simulink model "PulsePairProc_x4"  (Simulink 6.4)
settings: Solver=ode45  StartTime=0.0  StopTime=40000/12e6  RelTol=1e-3
libraries: xbsIndex_r4 x1049, simulink x4, dspsrcs4 x1
(part 3 of 8)

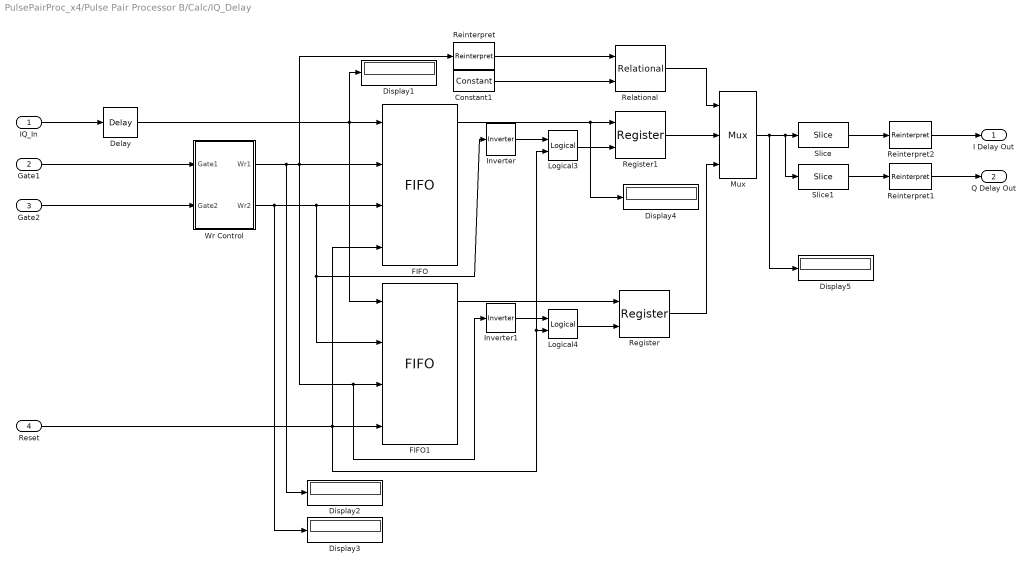
== system PulsePairProc_x4/Pulse Pair Processor B/Calc/IQ_Delay ==
  IQ_In : Inport
  Gate1 : Inport  Port=2
  Gate2 : Inport  Port=3
  Reset : Inport  Port=4
  Constant1 : xbsIndex_r4/Constant  arith_type=Unsigned  const=1  n_bits=1  bin_pt=0  explicit_period=off  period=1  equ=P=C  opselect=C  inp2=PCIN>>17  opr=+  inp1=P  carry=CIN  dbl_ovrd=off  block_type=constant
      settings: block_version=8.2
  Delay : xbsIndex_r4/Delay  en=off  latency=2  dbl_ovrd=off  reg_retiming=off  block_type=delay
      settings: infoedit=Hardware notes: A delay line is a chain, each link of which is an SRL16 followed by a flip-flop. If register retiming is enabled, the delay line is a chain of flip-flops.  block_version=8.2
  Display{1..5} (5 alike) : Display
  FIFO : xbsIndex_r4/FIFO  depth=1K  percent_nbits=1  rst=on  en=off  dbl_ovrd=off  mem_type=Block RAM  block_type=fifo
      settings: block_version=8.2
  FIFO1 : xbsIndex_r4/FIFO  depth=1K  percent_nbits=1  rst=on  en=off  dbl_ovrd=off  mem_type=Block RAM  block_type=fifo
      settings: block_version=8.2
  Inverter : xbsIndex_r4/Inverter  en=off  latency=1  dbl_ovrd=off  block_type=inv
      settings: block_version=8.2
  Inverter1 : xbsIndex_r4/Inverter  en=off  latency=1  dbl_ovrd=off  block_type=inv
      settings: block_version=8.2
  Logical3 : xbsIndex_r4/Logical  logical_function=OR  inputs=2  en=off  latency=0  precision=Full  arith_type=Unsigned  n_bits=16  bin_pt=0  align_bp=on  dbl_ovrd=off  block_type=logical
      settings: block_version=8.2
  Logical4 : xbsIndex_r4/Logical  logical_function=OR  inputs=2  en=off  latency=0  precision=Full  arith_type=Unsigned  n_bits=16  bin_pt=0  align_bp=on  dbl_ovrd=off  block_type=logical
      settings: block_version=8.2
  Mux : xbsIndex_r4/Mux  inputs=2  en=off  latency=0  precision=Full  arith_type=Unsigned  n_bits=16  bin_pt=14  quantization=Truncate  overflow=Wrap  dbl_ovrd=off  block_type=mux
      settings: block_version=8.2
  Register : xbsIndex_r4/Register  init=0  rst=on  en=off  dbl_ovrd=off  block_type=register
      settings: block_version=8.2
  Register1 : xbsIndex_r4/Register  init=0  rst=on  en=off  dbl_ovrd=off  block_type=register
      settings: block_version=8.2
  Reinterpret : xbsIndex_r4/Reinterpret  force_arith_type=on  arith_type=Unsigned  force_bin_pt=off  bin_pt=0  block_type=reinterpret
      settings: infoedit="Changes signal type without altering the binary representation.   You can changed the signal between signed and unsigned, and relocate the binary point.<P><P>Hardware notes: In hardware this block costs nothing.<P><P>Example:  Suppose the input is 6 bits wide, signed, with 2 fractional bits, and the output is forced to unsigned with 0 fractional bits.  Then an input of -2.0 (1110.00 in binary 2's complement) becomes an output of 56 (111000 in binary)."  block_version=8.2
  Reinterpret1 : xbsIndex_r4/Reinterpret  force_arith_type=on  arith_type="Signed  (2's comp)"  force_bin_pt=on  bin_pt=15  block_type=reinterpret
      settings: infoedit="Changes signal type without altering the binary representation.   You can changed the signal between signed and unsigned, and relocate the binary point.<P><P>Hardware notes: In hardware this block costs nothing.<P><P>Example:  Suppose the input is 6 bits wide, signed, with 2 fractional bits, and the output is forced to unsigned with 0 fractional bits.  Then an input of -2.0 (1110.00 in binary 2's complement) becomes an output of 56 (111000 in binary)."  block_version=8.2
  Reinterpret2 : xbsIndex_r4/Reinterpret  force_arith_type=on  arith_type="Signed  (2's comp)"  force_bin_pt=on  bin_pt=15  block_type=reinterpret
      settings: infoedit="Changes signal type without altering the binary representation.   You can changed the signal between signed and unsigned, and relocate the binary point.<P><P>Hardware notes: In hardware this block costs nothing.<P><P>Example:  Suppose the input is 6 bits wide, signed, with 2 fractional bits, and the output is forced to unsigned with 0 fractional bits.  Then an input of -2.0 (1110.00 in binary 2's complement) becomes an output of 56 (111000 in binary)."  block_version=8.2
  Relational : xbsIndex_r4/Relational  mode=a=b  en=off  latency=2  dbl_ovrd=off  block_type=relational
      settings: block_version=8.2
  Slice : xbsIndex_r4/Slice  nbits=16  boolean_output=off  mode=Upper Bit Location + Width  bit1=0  base1=MSB of Input  bit0=0  base0=LSB of Input  dbl_ovrd=off  block_type=slice
      settings: infoedit="Extracts a given range of bits from each input sample and presents it at the output.  The output type is ordinarily unsigned with binary point at zero, but can be Boolean when the slice is one bit wide.<P><P>Hardware notes: In hardware this block costs nothing."  block_version=8.2
  Slice1 : xbsIndex_r4/Slice  nbits=16  boolean_output=off  mode=Lower Bit Location + Width  bit1=0  base1=MSB of Input  bit0=0  base0=LSB of Input  dbl_ovrd=off  block_type=slice
      settings: infoedit="Extracts a given range of bits from each input sample and presents it at the output.  The output type is ordinarily unsigned with binary point at zero, but can be Boolean when the slice is one bit wide.<P><P>Hardware notes: In hardware this block costs nothing."  block_version=8.2
  Wr Control : Subsystem
  I Delay Out : Outport
  Q Delay Out : Outport  Port=2
  wires:
  IQ_In/1 -> Delay/1
  Reset/1 -> FIFO/4, FIFO1/4, Logical4/2, Logical3/2
  FIFO1/1 -> Register/1
  FIFO/1 -> Register1/1, Display4/1
  Register1/1 -> Mux/2
  Register/1 -> Mux/3
  Relational/1 -> Mux/1
  Constant1/1 -> Relational/2
  Reinterpret/1 -> Relational/1
  Delay/1 -> FIFO1/1, FIFO/1, Display1/1
  Logical3/1 -> Register1/2
  Logical4/1 -> Register/2
  Inverter1/1 -> Logical4/1
  Inverter/1 -> Logical3/1
  Mux/1 -> Slice/1, Slice1/1, Display5/1
  Slice/1 -> Reinterpret2/1
  Slice1/1 -> Reinterpret1/1
  Reinterpret1/1 -> Q Delay Out/1
  Reinterpret2/1 -> I Delay Out/1
  Wr Control/1(Wr1) -> FIFO/2, Reinterpret/1, FIFO1/3, Inverter1/1, Display2/1
  Wr Control/2(Wr2) -> FIFO/3, FIFO1/2, Inverter/1, Display3/1
  Gate1/1 -> Wr Control/1(Gate1)
  Gate2/1 -> Wr Control/2(Gate2)

== system PulsePairProc_x4/Pulse Pair Processor B/Calc/I^2+Q^2 ==
  I : Inport
  Q : Inport  Port=2
  AddSub : xbsIndex_r4/AddSub  mode=Addition  use_carryin=off  use_carryout=off  en=off  latency=1  precision=User Defined  arith_type=Unsigned  n_bits=32  bin_pt=32  quantization="Round  (unbiased: +/- Inf)"  overflow=Flag as error  dbl_ovrd=off  use_behavioral_HDL=off  pipelined=on  use_rpm=on  block_type=addsub
      settings: block_version=8.2
  Mult : xbsIndex_r4/Mult  precision=User Defined  arith_type=Unsigned  n_bits=32  bin_pt=32  quantization="Round  (unbiased: +/- Inf)"  overflow=Flag as error  en=off  latency=1  dbl_ovrd=off  use_behavioral_HDL=off  use_embedded=on  optimum_pipeline=off  use_rpm=on  placement_style=Rectangular shape  pipeline=on  block_type=mult
      settings: infoedit=Hardware notes: To use the internal pipeline stage of the dedicated multiplier you must select 'Pipeline for maximum performance'.  block_version=8.2
  Mult1 : xbsIndex_r4/Mult  precision=User Defined  arith_type=Unsigned  n_bits=32  bin_pt=32  quantization="Round  (unbiased: +/- Inf)"  overflow=Flag as error  en=off  latency=1  dbl_ovrd=off  use_behavioral_HDL=off  use_embedded=on  optimum_pipeline=off  use_rpm=on  placement_style=Rectangular shape  pipeline=on  block_type=mult
      settings: infoedit=Hardware notes: To use the internal pipeline stage of the dedicated multiplier you must select 'Pipeline for maximum performance'.  block_version=8.2
  P : Outport
  wires:
  Mult/1 -> AddSub/1
  Mult1/1 -> AddSub/2
  I/1 -> Mult/1, Mult/2
  Q/1 -> Mult1/1, Mult1/2
  AddSub/1 -> P/1

== system PulsePairProc_x4/Pulse Pair Processor B/Calc/Q*Id1-I*Qd1 ==
  Q : Inport
  I Delay 1 : Inport  Port=2
  I : Inport  Port=3
  Q Delay 1 : Inport  Port=4
  AddSub2 : xbsIndex_r4/AddSub  mode=Subtraction  use_carryin=off  use_carryout=off  en=off  latency=1  precision=User Defined  arith_type="Signed  (2's comp)"  n_bits=32  bin_pt=31  quantization="Round  (unbiased: +/- Inf)"  overflow=Flag as error  dbl_ovrd=off  use_behavioral_HDL=off  pipelined=on  use_rpm=on  block_type=addsub
      settings: block_version=8.2
  Mult4 : xbsIndex_r4/Mult  precision=User Defined  arith_type="Signed  (2's comp)"  n_bits=32  bin_pt=31  quantization="Round  (unbiased: +/- Inf)"  overflow=Saturate  en=off  latency=1  dbl_ovrd=off  use_behavioral_HDL=off  use_embedded=on  optimum_pipeline=off  use_rpm=on  placement_style=Rectangular shape  pipeline=on  block_type=mult
      settings: infoedit=Hardware notes: To use the internal pipeline stage of the dedicated multiplier you must select 'Pipeline for maximum performance'.  block_version=8.2
  Mult5 : xbsIndex_r4/Mult  precision=User Defined  arith_type="Signed  (2's comp)"  n_bits=32  bin_pt=31  quantization="Round  (unbiased: +/- Inf)"  overflow=Saturate  en=off  latency=1  dbl_ovrd=off  use_behavioral_HDL=off  use_embedded=on  optimum_pipeline=off  use_rpm=on  placement_style=Rectangular shape  pipeline=on  block_type=mult
      settings: infoedit=Hardware notes: To use the internal pipeline stage of the dedicated multiplier you must select 'Pipeline for maximum performance'.  block_version=8.2
  B : Outport
  wires:
  Mult4/1 -> AddSub2/1
  Mult5/1 -> AddSub2/2
  Q/1 -> Mult4/1
  I Delay 1/1 -> Mult4/2
  AddSub2/1 -> B/1
  I/1 -> Mult5/1
  Q Delay 1/1 -> Mult5/2

== system PulsePairProc_x4/Pulse Pair Processor B/Sum/A Avg ==
  A_Data_In : Inport
  M : Inport  Port=2
  N : Inport  Port=3
  Gate 1 : Inport  Port=4
  Gate 2 : Inport  Port=5
  Reset : Inport  Port=6
  Avg. A 1 : Subsystem
  Avg. A 2 : Subsystem
  A1 : Outport
  A2 : Outport  Port=2
  ABP G1 : Outport  Port=3
  ABP G2 : Outport  Port=4
  wires:
  A_Data_In/1 -> Avg. A 1/1(In), Avg. A 2/1(In)
  M/1 -> Avg. A 1/2(M), Avg. A 2/2(M)
  N/1 -> Avg. A 1/3(N), Avg. A 2/3(N)
  Avg. A 1/1(Out) -> A1/1
  Gate 1/1 -> Avg. A 1/4(Gate)
  Avg. A 2/1(Out) -> A2/1
  Gate 2/1 -> Avg. A 2/4(Gate)
  Avg. A 1/2(A,B,P Gate 1) -> ABP G1/1
  Avg. A 2/2(A,B,P Gate 1) -> ABP G2/1
  Reset/1 -> Avg. A 1/5(Reset), Avg. A 2/5(Reset)

== system PulsePairProc_x4/Pulse Pair Processor B/Sum/B Avg ==
  B_Data_In : Inport
  M : Inport  Port=2
  N : Inport  Port=3
  Gate 1 : Inport  Port=4
  Gate 2 : Inport  Port=5
  Reset : Inport  Port=6
  Avg. B 1 : Subsystem
  Avg. B 2 : Subsystem
  B1 : Outport
  B2 : Outport  Port=2
  wires:
  B_Data_In/1 -> Avg. B 1/1(In), Avg. B 2/1(In)
  M/1 -> Avg. B 1/2(M), Avg. B 2/2(M)
  N/1 -> Avg. B 1/3(N), Avg. B 2/3(N)
  Avg. B 1/1(Out) -> B1/1
  Gate 1/1 -> Avg. B 1/4(Gate)
  Avg. B 2/1(Out) -> B2/1
  Gate 2/1 -> Avg. B 2/4(Gate)
  Reset/1 -> Avg. B 1/5(Reset), Avg. B 2/5(Reset)

== system PulsePairProc_x4/Pulse Pair Processor B/Sum/Error Check ==
  Gate_1_In : Inport
  Gate_2_In : Inport  Port=2
  M_Reg : Inport  Port=3
  Counter : xbsIndex_r4/Counter  cnt_type=Free Running  cnt_to=Inf  operation=Up  start_count=0  cnt_by_val=1  arith_type=Unsigned  n_bits=10  bin_pt=0  load_pin=off  rst=on  en=on  explicit_period=on  period=1/12e6  dbl_ovrd=off  use_behavioral_HDL=off  use_rpm=off  block_type=counter
      settings: block_version=8.2
  Counter1 : xbsIndex_r4/Counter  cnt_type=Free Running  cnt_to=Inf  operation=Up  start_count=0  cnt_by_val=1  arith_type=Unsigned  n_bits=10  bin_pt=0  load_pin=off  rst=on  en=on  explicit_period=on  period=1/12e6  dbl_ovrd=off  use_behavioral_HDL=off  use_rpm=off  block_type=counter
      settings: block_version=8.2
  Delay{,1..3} (4 alike) : xbsIndex_r4/Delay  en=off  latency=1  dbl_ovrd=off  reg_retiming=off  block_type=delay
      settings: infoedit=Hardware notes: A delay line is a chain, each link of which is an SRL16 followed by a flip-flop. If register retiming is enabled, the delay line is a chain of flip-flops.  block_version=8.2
  Inverter : xbsIndex_r4/Inverter  en=off  latency=0  dbl_ovrd=off  block_type=inv
      settings: block_version=8.2
  Inverter1 : xbsIndex_r4/Inverter  en=off  latency=0  dbl_ovrd=off  block_type=inv
      settings: block_version=8.2
  Logical : xbsIndex_r4/Logical  logical_function=OR  inputs=2  en=off  latency=0  precision=Full  arith_type=Unsigned  n_bits=16  bin_pt=0  align_bp=on  dbl_ovrd=off  block_type=logical
      settings: block_version=8.2
  Register : xbsIndex_r4/Register  init=0  rst=off  en=on  dbl_ovrd=off  block_type=register
      settings: block_version=8.2
  Register1 : xbsIndex_r4/Register  init=0  rst=on  en=on  dbl_ovrd=off  block_type=register
      settings: block_version=8.2
  Register2 : xbsIndex_r4/Register  init=0  rst=off  en=on  dbl_ovrd=off  block_type=register
      settings: block_version=8.2
  Register3 : xbsIndex_r4/Register  init=0  rst=on  en=on  dbl_ovrd=off  block_type=register
      settings: block_version=8.2
  Relational : xbsIndex_r4/Relational  mode=a!=b  en=on  latency=1  dbl_ovrd=off  block_type=relational
      settings: block_version=8.2
  Relational1 : xbsIndex_r4/Relational  mode=a!=b  en=on  latency=1  dbl_ovrd=off  block_type=relational
      settings: block_version=8.2
  Sync Error : Outport
  wires:
  Inverter/1 -> Counter/1, Register/2, Delay/1, Register1/1
  Counter/1 -> Register/1
  Register/1 -> Relational/1
  Gate_1_In/1 -> Inverter/1, Counter/2, Delay1/1
  Delay/1 -> Register1/2
  Register1/1 -> Relational/3
  Delay1/1 -> Register1/3
  Inverter1/1 -> Counter1/1, Register2/2, Delay2/1, Register3/1
  Counter1/1 -> Register2/1
  Register2/1 -> Relational1/1
  Gate_2_In/1 -> Inverter1/1, Counter1/2, Delay3/1
  M_Reg/1 -> Relational1/2, Relational/2
  Delay2/1 -> Register3/2
  Register3/1 -> Relational1/3
  Delay3/1 -> Register3/3
  Relational/1 -> Logical/1
  Relational1/1 -> Logical/2
  Logical/1 -> Sync Error/1

== system PulsePairProc_x4/Pulse Pair Processor B/Sum/IQ Selector ==
  IQ Data : Inport
  IQ Gate 1 : Inport  Port=2
  IQ Gate 2 : Inport  Port=3
  IQ Index : Inport  Port=4
  IQ Length : Inport  Port=5
  Counter : xbsIndex_r4/Counter  cnt_type=Count Limited  cnt_to=1023  operation=Up  start_count=0  cnt_by_val=1  arith_type=Unsigned  n_bits=10  bin_pt=0  load_pin=off  rst=on  en=on  explicit_period=on  period=1/12e6  dbl_ovrd=off  use_behavioral_HDL=off  use_rpm=off  block_type=counter
      settings: block_version=8.2
  Counter1 : xbsIndex_r4/Counter  cnt_type=Count Limited  cnt_to=1023  operation=Up  start_count=0  cnt_by_val=1  arith_type=Unsigned  n_bits=10  bin_pt=0  load_pin=off  rst=on  en=on  explicit_period=on  period=1/12e6  dbl_ovrd=off  use_behavioral_HDL=off  use_rpm=off  block_type=counter
      settings: block_version=8.2
  Delay{,1..3} (4 alike) : xbsIndex_r4/Delay  en=off  latency=3  dbl_ovrd=off  reg_retiming=off  block_type=delay
      settings: infoedit=Hardware notes: A delay line is a chain, each link of which is an SRL16 followed by a flip-flop. If register retiming is enabled, the delay line is a chain of flip-flops.  block_version=8.2
  Inverter : xbsIndex_r4/Inverter  en=off  latency=0  dbl_ovrd=off  block_type=inv
      settings: block_version=8.2
  Inverter1 : xbsIndex_r4/Inverter  en=off  latency=0  dbl_ovrd=off  block_type=inv
      settings: block_version=8.2
  Inverter2 : xbsIndex_r4/Inverter  en=off  latency=0  dbl_ovrd=off  block_type=inv
      settings: block_version=8.2
  Inverter4 : xbsIndex_r4/Inverter  en=off  latency=1  dbl_ovrd=off  block_type=inv
      settings: block_version=8.2
  Logical{,1..3} (4 alike) : xbsIndex_r4/Logical  logical_function=OR  inputs=2  en=off  latency=0  precision=Full  arith_type=Unsigned  n_bits=16  bin_pt=0  align_bp=on  dbl_ovrd=off  block_type=logical
      settings: block_version=8.2
  Logical4 : xbsIndex_r4/Logical  logical_function=AND  inputs=2  en=off  latency=0  precision=Full  arith_type=Unsigned  n_bits=16  bin_pt=0  align_bp=on  dbl_ovrd=off  block_type=logical
      settings: block_version=8.2
  Logical5 : xbsIndex_r4/Logical  logical_function=AND  inputs=2  en=off  latency=0  precision=Full  arith_type=Unsigned  n_bits=16  bin_pt=0  align_bp=on  dbl_ovrd=off  block_type=logical
      settings: block_version=8.2
  Register1 : xbsIndex_r4/Register  init=0  rst=on  en=off  dbl_ovrd=off  block_type=register
      settings: block_version=8.2
  Relational : xbsIndex_r4/Relational  mode=a>b  en=on  latency=1  dbl_ovrd=off  block_type=relational
      settings: block_version=8.2
  Relational1 : xbsIndex_r4/Relational  mode=a<b  en=on  latency=1  dbl_ovrd=off  block_type=relational
      settings: block_version=8.2
  IQ Out : Outport
  IQ Gate 1 Out : Outport  Port=2
  IQ Gate 2 Out : Outport  Port=3
  wires:
  Counter/1 -> Relational/1
  IQ Index/1 -> Relational/2
  Inverter/1 -> Counter/1, Delay/1
  Inverter1/1 -> Counter1/1
  Relational/1 -> Inverter1/1, Counter1/2, Relational1/3
  Counter1/1 -> Relational1/1
  Relational1/1 -> Inverter2/1
  IQ Data/1 -> Register1/1
  Register1/1 -> Delay2/1
  Logical/1 -> Inverter/1, Counter/2, Relational/3
  IQ Gate 2/1 -> Logical/2, Logical5/2
  IQ Gate 1/1 -> Logical/1, Logical4/2
  Logical1/1 -> Register1/2, Inverter4/1
  Inverter2/1 -> Logical1/2
  Delay/1 -> Logical1/1
  IQ Length/1 -> Relational1/2
  Logical2/1 -> IQ Gate 1 Out/1
  Delay1/1 -> Logical2/1
  Delay2/1 -> IQ Out/1
  Inverter4/1 -> Logical4/1, Logical5/1
  Logical4/1 -> Delay1/1, Logical2/2
  Logical3/1 -> IQ Gate 2 Out/1
  Delay3/1 -> Logical3/1
  Logical5/1 -> Delay3/1, Logical3/2

== system PulsePairProc_x4/Pulse Pair Processor B/Sum/P Avg ==
  P_Data_In : Inport
  M : Inport  Port=2
  N : Inport  Port=3
  Gate 1 : Inport  Port=4
  Gate 2 : Inport  Port=5
  Reset : Inport  Port=6
  Avg. P 1 : Subsystem
  Avg. P 2 : Subsystem
  P1 : Outport
  P2 : Outport  Port=2
  wires:
  P_Data_In/1 -> Avg. P 1/1(In), Avg. P 2/1(In)
  M/1 -> Avg. P 1/2(M), Avg. P 2/2(M)
  N/1 -> Avg. P 1/3(N), Avg. P 2/3(N)
  Avg. P 1/1(Out) -> P1/1
  Gate 1/1 -> Avg. P 1/4(Gate)
  Avg. P 2/1(Out) -> P2/1
  Gate 2/1 -> Avg. P 2/4(Gate)
  Reset/1 -> Avg. P 1/5(Reset), Avg. P 2/5(Reset)

== system PulsePairProc_x4/Pulse Pair Processor C/Calc/I*Id1+Q*Qd1 ==
  I : Inport
  I Delay 1 : Inport  Port=2
  Q : Inport  Port=3
  Q Delay 1 : Inport  Port=4
  AddSub1 : xbsIndex_r4/AddSub  mode=Addition  use_carryin=off  use_carryout=off  en=off  latency=1  precision=User Defined  arith_type="Signed  (2's comp)"  n_bits=32  bin_pt=31  quantization="Round  (unbiased: +/- Inf)"  overflow=Flag as error  dbl_ovrd=off  use_behavioral_HDL=off  pipelined=on  use_rpm=on  block_type=addsub
      settings: block_version=8.2
  Mult2 : xbsIndex_r4/Mult  precision=User Defined  arith_type="Signed  (2's comp)"  n_bits=32  bin_pt=31  quantization="Round  (unbiased: +/- Inf)"  overflow=Saturate  en=off  latency=1  dbl_ovrd=off  use_behavioral_HDL=off  use_embedded=on  optimum_pipeline=off  use_rpm=on  placement_style=Rectangular shape  pipeline=on  block_type=mult
      settings: infoedit=Hardware notes: To use the internal pipeline stage of the dedicated multiplier you must select 'Pipeline for maximum performance'.  block_version=8.2
  Mult3 : xbsIndex_r4/Mult  precision=User Defined  arith_type="Signed  (2's comp)"  n_bits=32  bin_pt=31  quantization="Round  (unbiased: +/- Inf)"  overflow=Saturate  en=off  latency=1  dbl_ovrd=off  use_behavioral_HDL=off  use_embedded=on  optimum_pipeline=off  use_rpm=on  placement_style=Rectangular shape  pipeline=on  block_type=mult
      settings: infoedit=Hardware notes: To use the internal pipeline stage of the dedicated multiplier you must select 'Pipeline for maximum performance'.  block_version=8.2
  A : Outport
  wires:
  Mult2/1 -> AddSub1/1
  Mult3/1 -> AddSub1/2
  I/1 -> Mult2/1
  I Delay 1/1 -> Mult2/2
  AddSub1/1 -> A/1
  Q/1 -> Mult3/1
  Q Delay 1/1 -> Mult3/2

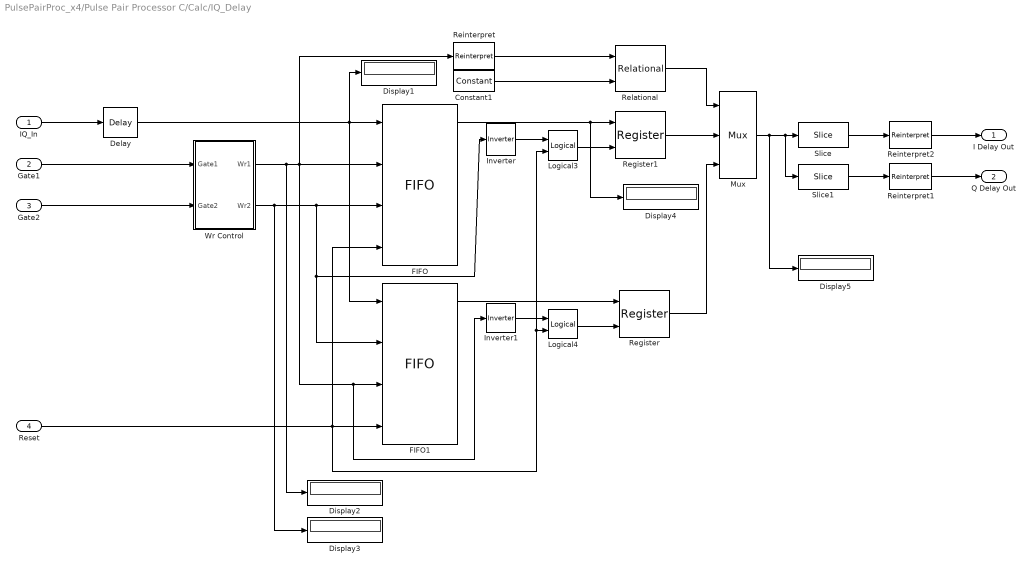
== system PulsePairProc_x4/Pulse Pair Processor C/Calc/IQ_Delay ==
  IQ_In : Inport
  Gate1 : Inport  Port=2
  Gate2 : Inport  Port=3
  Reset : Inport  Port=4
  Constant1 : xbsIndex_r4/Constant  arith_type=Unsigned  const=1  n_bits=1  bin_pt=0  explicit_period=off  period=1  equ=P=C  opselect=C  inp2=PCIN>>17  opr=+  inp1=P  carry=CIN  dbl_ovrd=off  block_type=constant
      settings: block_version=8.2
  Delay : xbsIndex_r4/Delay  en=off  latency=2  dbl_ovrd=off  reg_retiming=off  block_type=delay
      settings: infoedit=Hardware notes: A delay line is a chain, each link of which is an SRL16 followed by a flip-flop. If register retiming is enabled, the delay line is a chain of flip-flops.  block_version=8.2
  Display{1..5} (5 alike) : Display
  FIFO : xbsIndex_r4/FIFO  depth=1K  percent_nbits=1  rst=on  en=off  dbl_ovrd=off  mem_type=Block RAM  block_type=fifo
      settings: block_version=8.2
  FIFO1 : xbsIndex_r4/FIFO  depth=1K  percent_nbits=1  rst=on  en=off  dbl_ovrd=off  mem_type=Block RAM  block_type=fifo
      settings: block_version=8.2
  Inverter : xbsIndex_r4/Inverter  en=off  latency=1  dbl_ovrd=off  block_type=inv
      settings: block_version=8.2
  Inverter1 : xbsIndex_r4/Inverter  en=off  latency=1  dbl_ovrd=off  block_type=inv
      settings: block_version=8.2
  Logical3 : xbsIndex_r4/Logical  logical_function=OR  inputs=2  en=off  latency=0  precision=Full  arith_type=Unsigned  n_bits=16  bin_pt=0  align_bp=on  dbl_ovrd=off  block_type=logical
      settings: block_version=8.2
  Logical4 : xbsIndex_r4/Logical  logical_function=OR  inputs=2  en=off  latency=0  precision=Full  arith_type=Unsigned  n_bits=16  bin_pt=0  align_bp=on  dbl_ovrd=off  block_type=logical
      settings: block_version=8.2
  Mux : xbsIndex_r4/Mux  inputs=2  en=off  latency=0  precision=Full  arith_type=Unsigned  n_bits=16  bin_pt=14  quantization=Truncate  overflow=Wrap  dbl_ovrd=off  block_type=mux
      settings: block_version=8.2
  Register : xbsIndex_r4/Register  init=0  rst=on  en=off  dbl_ovrd=off  block_type=register
      settings: block_version=8.2
  Register1 : xbsIndex_r4/Register  init=0  rst=on  en=off  dbl_ovrd=off  block_type=register
      settings: block_version=8.2
  Reinterpret : xbsIndex_r4/Reinterpret  force_arith_type=on  arith_type=Unsigned  force_bin_pt=off  bin_pt=0  block_type=reinterpret
      settings: infoedit="Changes signal type without altering the binary representation.   You can changed the signal between signed and unsigned, and relocate the binary point.<P><P>Hardware notes: In hardware this block costs nothing.<P><P>Example:  Suppose the input is 6 bits wide, signed, with 2 fractional bits, and the output is forced to unsigned with 0 fractional bits.  Then an input of -2.0 (1110.00 in binary 2's complement) becomes an output of 56 (111000 in binary)."  block_version=8.2
  Reinterpret1 : xbsIndex_r4/Reinterpret  force_arith_type=on  arith_type="Signed  (2's comp)"  force_bin_pt=on  bin_pt=15  block_type=reinterpret
      settings: infoedit="Changes signal type without altering the binary representation.   You can changed the signal between signed and unsigned, and relocate the binary point.<P><P>Hardware notes: In hardware this block costs nothing.<P><P>Example:  Suppose the input is 6 bits wide, signed, with 2 fractional bits, and the output is forced to unsigned with 0 fractional bits.  Then an input of -2.0 (1110.00 in binary 2's complement) becomes an output of 56 (111000 in binary)."  block_version=8.2
  Reinterpret2 : xbsIndex_r4/Reinterpret  force_arith_type=on  arith_type="Signed  (2's comp)"  force_bin_pt=on  bin_pt=15  block_type=reinterpret
      settings: infoedit="Changes signal type without altering the binary representation.   You can changed the signal between signed and unsigned, and relocate the binary point.<P><P>Hardware notes: In hardware this block costs nothing.<P><P>Example:  Suppose the input is 6 bits wide, signed, with 2 fractional bits, and the output is forced to unsigned with 0 fractional bits.  Then an input of -2.0 (1110.00 in binary 2's complement) becomes an output of 56 (111000 in binary)."  block_version=8.2
  Relational : xbsIndex_r4/Relational  mode=a=b  en=off  latency=2  dbl_ovrd=off  block_type=relational
      settings: block_version=8.2
  Slice : xbsIndex_r4/Slice  nbits=16  boolean_output=off  mode=Upper Bit Location + Width  bit1=0  base1=MSB of Input  bit0=0  base0=LSB of Input  dbl_ovrd=off  block_type=slice
      settings: infoedit="Extracts a given range of bits from each input sample and presents it at the output.  The output type is ordinarily unsigned with binary point at zero, but can be Boolean when the slice is one bit wide.<P><P>Hardware notes: In hardware this block costs nothing."  block_version=8.2
  Slice1 : xbsIndex_r4/Slice  nbits=16  boolean_output=off  mode=Lower Bit Location + Width  bit1=0  base1=MSB of Input  bit0=0  base0=LSB of Input  dbl_ovrd=off  block_type=slice
      settings: infoedit="Extracts a given range of bits from each input sample and presents it at the output.  The output type is ordinarily unsigned with binary point at zero, but can be Boolean when the slice is one bit wide.<P><P>Hardware notes: In hardware this block costs nothing."  block_version=8.2
  Wr Control : Subsystem
  I Delay Out : Outport
  Q Delay Out : Outport  Port=2
  wires:
  IQ_In/1 -> Delay/1
  Reset/1 -> FIFO/4, FIFO1/4, Logical4/2, Logical3/2
  FIFO1/1 -> Register/1
  FIFO/1 -> Register1/1, Display4/1
  Register1/1 -> Mux/2
  Register/1 -> Mux/3
  Relational/1 -> Mux/1
  Constant1/1 -> Relational/2
  Reinterpret/1 -> Relational/1
  Delay/1 -> FIFO1/1, FIFO/1, Display1/1
  Logical3/1 -> Register1/2
  Logical4/1 -> Register/2
  Inverter1/1 -> Logical4/1
  Inverter/1 -> Logical3/1
  Mux/1 -> Slice/1, Slice1/1, Display5/1
  Slice/1 -> Reinterpret2/1
  Slice1/1 -> Reinterpret1/1
  Reinterpret1/1 -> Q Delay Out/1
  Reinterpret2/1 -> I Delay Out/1
  Wr Control/1(Wr1) -> FIFO/2, Reinterpret/1, FIFO1/3, Inverter1/1, Display2/1
  Wr Control/2(Wr2) -> FIFO/3, FIFO1/2, Inverter/1, Display3/1
  Gate1/1 -> Wr Control/1(Gate1)
  Gate2/1 -> Wr Control/2(Gate2)

== system PulsePairProc_x4/Pulse Pair Processor C/Calc/I^2+Q^2 ==
  I : Inport
  Q : Inport  Port=2
  AddSub : xbsIndex_r4/AddSub  mode=Addition  use_carryin=off  use_carryout=off  en=off  latency=1  precision=User Defined  arith_type=Unsigned  n_bits=32  bin_pt=32  quantization="Round  (unbiased: +/- Inf)"  overflow=Flag as error  dbl_ovrd=off  use_behavioral_HDL=off  pipelined=on  use_rpm=on  block_type=addsub
      settings: block_version=8.2
  Mult : xbsIndex_r4/Mult  precision=User Defined  arith_type=Unsigned  n_bits=32  bin_pt=32  quantization="Round  (unbiased: +/- Inf)"  overflow=Flag as error  en=off  latency=1  dbl_ovrd=off  use_behavioral_HDL=off  use_embedded=on  optimum_pipeline=off  use_rpm=on  placement_style=Rectangular shape  pipeline=on  block_type=mult
      settings: infoedit=Hardware notes: To use the internal pipeline stage of the dedicated multiplier you must select 'Pipeline for maximum performance'.  block_version=8.2
  Mult1 : xbsIndex_r4/Mult  precision=User Defined  arith_type=Unsigned  n_bits=32  bin_pt=32  quantization="Round  (unbiased: +/- Inf)"  overflow=Flag as error  en=off  latency=1  dbl_ovrd=off  use_behavioral_HDL=off  use_embedded=on  optimum_pipeline=off  use_rpm=on  placement_style=Rectangular shape  pipeline=on  block_type=mult
      settings: infoedit=Hardware notes: To use the internal pipeline stage of the dedicated multiplier you must select 'Pipeline for maximum performance'.  block_version=8.2
  P : Outport
  wires:
  Mult/1 -> AddSub/1
  Mult1/1 -> AddSub/2
  I/1 -> Mult/1, Mult/2
  Q/1 -> Mult1/1, Mult1/2
  AddSub/1 -> P/1

== system PulsePairProc_x4/Pulse Pair Processor C/Calc/Q*Id1-I*Qd1 ==
  Q : Inport
  I Delay 1 : Inport  Port=2
  I : Inport  Port=3
  Q Delay 1 : Inport  Port=4
  AddSub2 : xbsIndex_r4/AddSub  mode=Subtraction  use_carryin=off  use_carryout=off  en=off  latency=1  precision=User Defined  arith_type="Signed  (2's comp)"  n_bits=32  bin_pt=31  quantization="Round  (unbiased: +/- Inf)"  overflow=Flag as error  dbl_ovrd=off  use_behavioral_HDL=off  pipelined=on  use_rpm=on  block_type=addsub
      settings: block_version=8.2
  Mult4 : xbsIndex_r4/Mult  precision=User Defined  arith_type="Signed  (2's comp)"  n_bits=32  bin_pt=31  quantization="Round  (unbiased: +/- Inf)"  overflow=Saturate  en=off  latency=1  dbl_ovrd=off  use_behavioral_HDL=off  use_embedded=on  optimum_pipeline=off  use_rpm=on  placement_style=Rectangular shape  pipeline=on  block_type=mult
      settings: infoedit=Hardware notes: To use the internal pipeline stage of the dedicated multiplier you must select 'Pipeline for maximum performance'.  block_version=8.2
  Mult5 : xbsIndex_r4/Mult  precision=User Defined  arith_type="Signed  (2's comp)"  n_bits=32  bin_pt=31  quantization="Round  (unbiased: +/- Inf)"  overflow=Saturate  en=off  latency=1  dbl_ovrd=off  use_behavioral_HDL=off  use_embedded=on  optimum_pipeline=off  use_rpm=on  placement_style=Rectangular shape  pipeline=on  block_type=mult
      settings: infoedit=Hardware notes: To use the internal pipeline stage of the dedicated multiplier you must select 'Pipeline for maximum performance'.  block_version=8.2
  B : Outport
  wires:
  Mult4/1 -> AddSub2/1
  Mult5/1 -> AddSub2/2
  Q/1 -> Mult4/1
  I Delay 1/1 -> Mult4/2
  AddSub2/1 -> B/1
  I/1 -> Mult5/1
  Q Delay 1/1 -> Mult5/2

== system PulsePairProc_x4/Pulse Pair Processor C/Sum/A Avg ==
  A_Data_In : Inport
  M : Inport  Port=2
  N : Inport  Port=3
  Gate 1 : Inport  Port=4
  Gate 2 : Inport  Port=5
  Reset : Inport  Port=6
  Avg. A 1 : Subsystem
  Avg. A 2 : Subsystem
  A1 : Outport
  A2 : Outport  Port=2
  ABP G1 : Outport  Port=3
  ABP G2 : Outport  Port=4
  wires:
  A_Data_In/1 -> Avg. A 1/1(In), Avg. A 2/1(In)
  M/1 -> Avg. A 1/2(M), Avg. A 2/2(M)
  N/1 -> Avg. A 1/3(N), Avg. A 2/3(N)
  Avg. A 1/1(Out) -> A1/1
  Gate 1/1 -> Avg. A 1/4(Gate)
  Avg. A 2/1(Out) -> A2/1
  Gate 2/1 -> Avg. A 2/4(Gate)
  Avg. A 1/2(A,B,P Gate 1) -> ABP G1/1
  Avg. A 2/2(A,B,P Gate 1) -> ABP G2/1
  Reset/1 -> Avg. A 1/5(Reset), Avg. A 2/5(Reset)

== system PulsePairProc_x4/Pulse Pair Processor C/Sum/B Avg ==
  B_Data_In : Inport
  M : Inport  Port=2
  N : Inport  Port=3
  Gate 1 : Inport  Port=4
  Gate 2 : Inport  Port=5
  Reset : Inport  Port=6
  Avg. B 1 : Subsystem
  Avg. B 2 : Subsystem
  B1 : Outport
  B2 : Outport  Port=2
  wires:
  B_Data_In/1 -> Avg. B 1/1(In), Avg. B 2/1(In)
  M/1 -> Avg. B 1/2(M), Avg. B 2/2(M)
  N/1 -> Avg. B 1/3(N), Avg. B 2/3(N)
  Avg. B 1/1(Out) -> B1/1
  Gate 1/1 -> Avg. B 1/4(Gate)
  Avg. B 2/1(Out) -> B2/1
  Gate 2/1 -> Avg. B 2/4(Gate)
  Reset/1 -> Avg. B 1/5(Reset), Avg. B 2/5(Reset)

== system PulsePairProc_x4/Pulse Pair Processor C/Sum/Error Check ==
  Gate_1_In : Inport
  Gate_2_In : Inport  Port=2
  M_Reg : Inport  Port=3
  Counter : xbsIndex_r4/Counter  cnt_type=Free Running  cnt_to=Inf  operation=Up  start_count=0  cnt_by_val=1  arith_type=Unsigned  n_bits=10  bin_pt=0  load_pin=off  rst=on  en=on  explicit_period=on  period=1/12e6  dbl_ovrd=off  use_behavioral_HDL=off  use_rpm=off  block_type=counter
      settings: block_version=8.2
  Counter1 : xbsIndex_r4/Counter  cnt_type=Free Running  cnt_to=Inf  operation=Up  start_count=0  cnt_by_val=1  arith_type=Unsigned  n_bits=10  bin_pt=0  load_pin=off  rst=on  en=on  explicit_period=on  period=1/12e6  dbl_ovrd=off  use_behavioral_HDL=off  use_rpm=off  block_type=counter
      settings: block_version=8.2
  Delay{,1..3} (4 alike) : xbsIndex_r4/Delay  en=off  latency=1  dbl_ovrd=off  reg_retiming=off  block_type=delay
      settings: infoedit=Hardware notes: A delay line is a chain, each link of which is an SRL16 followed by a flip-flop. If register retiming is enabled, the delay line is a chain of flip-flops.  block_version=8.2
  Inverter : xbsIndex_r4/Inverter  en=off  latency=0  dbl_ovrd=off  block_type=inv
      settings: block_version=8.2
  Inverter1 : xbsIndex_r4/Inverter  en=off  latency=0  dbl_ovrd=off  block_type=inv
      settings: block_version=8.2
  Logical : xbsIndex_r4/Logical  logical_function=OR  inputs=2  en=off  latency=0  precision=Full  arith_type=Unsigned  n_bits=16  bin_pt=0  align_bp=on  dbl_ovrd=off  block_type=logical
      settings: block_version=8.2
  Register : xbsIndex_r4/Register  init=0  rst=off  en=on  dbl_ovrd=off  block_type=register
      settings: block_version=8.2
  Register1 : xbsIndex_r4/Register  init=0  rst=on  en=on  dbl_ovrd=off  block_type=register
      settings: block_version=8.2
  Register2 : xbsIndex_r4/Register  init=0  rst=off  en=on  dbl_ovrd=off  block_type=register
      settings: block_version=8.2
  Register3 : xbsIndex_r4/Register  init=0  rst=on  en=on  dbl_ovrd=off  block_type=register
      settings: block_version=8.2
  Relational : xbsIndex_r4/Relational  mode=a!=b  en=on  latency=1  dbl_ovrd=off  block_type=relational
      settings: block_version=8.2
  Relational1 : xbsIndex_r4/Relational  mode=a!=b  en=on  latency=1  dbl_ovrd=off  block_type=relational
      settings: block_version=8.2
  Sync Error : Outport
  wires:
  Inverter/1 -> Counter/1, Register/2, Delay/1, Register1/1
  Counter/1 -> Register/1
  Register/1 -> Relational/1
  Gate_1_In/1 -> Inverter/1, Counter/2, Delay1/1
  Delay/1 -> Register1/2
  Register1/1 -> Relational/3
  Delay1/1 -> Register1/3
  Inverter1/1 -> Counter1/1, Register2/2, Delay2/1, Register3/1
  Counter1/1 -> Register2/1
  Register2/1 -> Relational1/1
  Gate_2_In/1 -> Inverter1/1, Counter1/2, Delay3/1
  M_Reg/1 -> Relational1/2, Relational/2
  Delay2/1 -> Register3/2
  Register3/1 -> Relational1/3
  Delay3/1 -> Register3/3
  Relational/1 -> Logical/1
  Relational1/1 -> Logical/2
  Logical/1 -> Sync Error/1

== system PulsePairProc_x4/Pulse Pair Processor C/Sum/IQ Selector ==
  IQ Data : Inport
  IQ Gate 1 : Inport  Port=2
  IQ Gate 2 : Inport  Port=3
  IQ Index : Inport  Port=4
  IQ Length : Inport  Port=5
  Counter : xbsIndex_r4/Counter  cnt_type=Count Limited  cnt_to=1023  operation=Up  start_count=0  cnt_by_val=1  arith_type=Unsigned  n_bits=10  bin_pt=0  load_pin=off  rst=on  en=on  explicit_period=on  period=1/12e6  dbl_ovrd=off  use_behavioral_HDL=off  use_rpm=off  block_type=counter
      settings: block_version=8.2
  Counter1 : xbsIndex_r4/Counter  cnt_type=Count Limited  cnt_to=1023  operation=Up  start_count=0  cnt_by_val=1  arith_type=Unsigned  n_bits=10  bin_pt=0  load_pin=off  rst=on  en=on  explicit_period=on  period=1/12e6  dbl_ovrd=off  use_behavioral_HDL=off  use_rpm=off  block_type=counter
      settings: block_version=8.2
  Delay{,1..3} (4 alike) : xbsIndex_r4/Delay  en=off  latency=3  dbl_ovrd=off  reg_retiming=off  block_type=delay
      settings: infoedit=Hardware notes: A delay line is a chain, each link of which is an SRL16 followed by a flip-flop. If register retiming is enabled, the delay line is a chain of flip-flops.  block_version=8.2
  Inverter : xbsIndex_r4/Inverter  en=off  latency=0  dbl_ovrd=off  block_type=inv
      settings: block_version=8.2
  Inverter1 : xbsIndex_r4/Inverter  en=off  latency=0  dbl_ovrd=off  block_type=inv
      settings: block_version=8.2
  Inverter2 : xbsIndex_r4/Inverter  en=off  latency=0  dbl_ovrd=off  block_type=inv
      settings: block_version=8.2
  Inverter4 : xbsIndex_r4/Inverter  en=off  latency=1  dbl_ovrd=off  block_type=inv
      settings: block_version=8.2
  Logical{,1..3} (4 alike) : xbsIndex_r4/Logical  logical_function=OR  inputs=2  en=off  latency=0  precision=Full  arith_type=Unsigned  n_bits=16  bin_pt=0  align_bp=on  dbl_ovrd=off  block_type=logical
      settings: block_version=8.2
  Logical4 : xbsIndex_r4/Logical  logical_function=AND  inputs=2  en=off  latency=0  precision=Full  arith_type=Unsigned  n_bits=16  bin_pt=0  align_bp=on  dbl_ovrd=off  block_type=logical
      settings: block_version=8.2
  Logical5 : xbsIndex_r4/Logical  logical_function=AND  inputs=2  en=off  latency=0  precision=Full  arith_type=Unsigned  n_bits=16  bin_pt=0  align_bp=on  dbl_ovrd=off  block_type=logical
      settings: block_version=8.2
  Register1 : xbsIndex_r4/Register  init=0  rst=on  en=off  dbl_ovrd=off  block_type=register
      settings: block_version=8.2
  Relational : xbsIndex_r4/Relational  mode=a>b  en=on  latency=1  dbl_ovrd=off  block_type=relational
      settings: block_version=8.2
  Relational1 : xbsIndex_r4/Relational  mode=a<b  en=on  latency=1  dbl_ovrd=off  block_type=relational
      settings: block_version=8.2
  IQ Out : Outport
  IQ Gate 1 Out : Outport  Port=2
  IQ Gate 2 Out : Outport  Port=3
  wires:
  Counter/1 -> Relational/1
  IQ Index/1 -> Relational/2
  Inverter/1 -> Counter/1, Delay/1
  Inverter1/1 -> Counter1/1
  Relational/1 -> Inverter1/1, Counter1/2, Relational1/3
  Counter1/1 -> Relational1/1
  Relational1/1 -> Inverter2/1
  IQ Data/1 -> Register1/1
  Register1/1 -> Delay2/1
  Logical/1 -> Inverter/1, Counter/2, Relational/3
  IQ Gate 2/1 -> Logical/2, Logical5/2
  IQ Gate 1/1 -> Logical/1, Logical4/2
  Logical1/1 -> Register1/2, Inverter4/1
  Inverter2/1 -> Logical1/2
  Delay/1 -> Logical1/1
  IQ Length/1 -> Relational1/2
  Logical2/1 -> IQ Gate 1 Out/1
  Delay1/1 -> Logical2/1
  Delay2/1 -> IQ Out/1
  Inverter4/1 -> Logical4/1, Logical5/1
  Logical4/1 -> Delay1/1, Logical2/2
  Logical3/1 -> IQ Gate 2 Out/1
  Delay3/1 -> Logical3/1
  Logical5/1 -> Delay3/1, Logical3/2

== system PulsePairProc_x4/Pulse Pair Processor C/Sum/P Avg ==
  P_Data_In : Inport
  M : Inport  Port=2
  N : Inport  Port=3
  Gate 1 : Inport  Port=4
  Gate 2 : Inport  Port=5
  Reset : Inport  Port=6
  Avg. P 1 : Subsystem
  Avg. P 2 : Subsystem
  P1 : Outport
  P2 : Outport  Port=2
  wires:
  P_Data_In/1 -> Avg. P 1/1(In), Avg. P 2/1(In)
  M/1 -> Avg. P 1/2(M), Avg. P 2/2(M)
  N/1 -> Avg. P 1/3(N), Avg. P 2/3(N)
  Avg. P 1/1(Out) -> P1/1
  Gate 1/1 -> Avg. P 1/4(Gate)
  Avg. P 2/1(Out) -> P2/1
  Gate 2/1 -> Avg. P 2/4(Gate)
  Reset/1 -> Avg. P 1/5(Reset), Avg. P 2/5(Reset)

== system PulsePairProc_x4/Pulse Pair Processor D/Calc/I*Id1+Q*Qd1 ==
  I : Inport
  I Delay 1 : Inport  Port=2
  Q : Inport  Port=3
  Q Delay 1 : Inport  Port=4
  AddSub1 : xbsIndex_r4/AddSub  mode=Addition  use_carryin=off  use_carryout=off  en=off  latency=1  precision=User Defined  arith_type="Signed  (2's comp)"  n_bits=32  bin_pt=31  quantization="Round  (unbiased: +/- Inf)"  overflow=Flag as error  dbl_ovrd=off  use_behavioral_HDL=off  pipelined=on  use_rpm=on  block_type=addsub
      settings: block_version=8.2
  Mult2 : xbsIndex_r4/Mult  precision=User Defined  arith_type="Signed  (2's comp)"  n_bits=32  bin_pt=31  quantization="Round  (unbiased: +/- Inf)"  overflow=Saturate  en=off  latency=1  dbl_ovrd=off  use_behavioral_HDL=off  use_embedded=on  optimum_pipeline=off  use_rpm=on  placement_style=Rectangular shape  pipeline=on  block_type=mult
      settings: infoedit=Hardware notes: To use the internal pipeline stage of the dedicated multiplier you must select 'Pipeline for maximum performance'.  block_version=8.2
  Mult3 : xbsIndex_r4/Mult  precision=User Defined  arith_type="Signed  (2's comp)"  n_bits=32  bin_pt=31  quantization="Round  (unbiased: +/- Inf)"  overflow=Saturate  en=off  latency=1  dbl_ovrd=off  use_behavioral_HDL=off  use_embedded=on  optimum_pipeline=off  use_rpm=on  placement_style=Rectangular shape  pipeline=on  block_type=mult
      settings: infoedit=Hardware notes: To use the internal pipeline stage of the dedicated multiplier you must select 'Pipeline for maximum performance'.  block_version=8.2
  A : Outport
  wires:
  Mult2/1 -> AddSub1/1
  Mult3/1 -> AddSub1/2
  I/1 -> Mult2/1
  I Delay 1/1 -> Mult2/2
  AddSub1/1 -> A/1
  Q/1 -> Mult3/1
  Q Delay 1/1 -> Mult3/2

== system PulsePairProc_x4/Pulse Pair Processor D/Calc/IQ_Delay ==
  IQ_In : Inport
  Gate1 : Inport  Port=2
  Gate2 : Inport  Port=3
  Reset : Inport  Port=4
  Constant1 : xbsIndex_r4/Constant  arith_type=Unsigned  const=1  n_bits=1  bin_pt=0  explicit_period=off  period=1  equ=P=C  opselect=C  inp2=PCIN>>17  opr=+  inp1=P  carry=CIN  dbl_ovrd=off  block_type=constant
      settings: block_version=8.2
  Delay : xbsIndex_r4/Delay  en=off  latency=2  dbl_ovrd=off  reg_retiming=off  block_type=delay
      settings: infoedit=Hardware notes: A delay line is a chain, each link of which is an SRL16 followed by a flip-flop. If register retiming is enabled, the delay line is a chain of flip-flops.  block_version=8.2
  Display{1..5} (5 alike) : Display
  FIFO : xbsIndex_r4/FIFO  depth=1K  percent_nbits=1  rst=on  en=off  dbl_ovrd=off  mem_type=Block RAM  block_type=fifo
      settings: block_version=8.2
  FIFO1 : xbsIndex_r4/FIFO  depth=1K  percent_nbits=1  rst=on  en=off  dbl_ovrd=off  mem_type=Block RAM  block_type=fifo
      settings: block_version=8.2
  Inverter : xbsIndex_r4/Inverter  en=off  latency=1  dbl_ovrd=off  block_type=inv
      settings: block_version=8.2
  Inverter1 : xbsIndex_r4/Inverter  en=off  latency=1  dbl_ovrd=off  block_type=inv
      settings: block_version=8.2
  Logical3 : xbsIndex_r4/Logical  logical_function=OR  inputs=2  en=off  latency=0  precision=Full  arith_type=Unsigned  n_bits=16  bin_pt=0  align_bp=on  dbl_ovrd=off  block_type=logical
      settings: block_version=8.2
  Logical4 : xbsIndex_r4/Logical  logical_function=OR  inputs=2  en=off  latency=0  precision=Full  arith_type=Unsigned  n_bits=16  bin_pt=0  align_bp=on  dbl_ovrd=off  block_type=logical
      settings: block_version=8.2
  Mux : xbsIndex_r4/Mux  inputs=2  en=off  latency=0  precision=Full  arith_type=Unsigned  n_bits=16  bin_pt=14  quantization=Truncate  overflow=Wrap  dbl_ovrd=off  block_type=mux
      settings: block_version=8.2
  Register : xbsIndex_r4/Register  init=0  rst=on  en=off  dbl_ovrd=off  block_type=register
      settings: block_version=8.2
  Register1 : xbsIndex_r4/Register  init=0  rst=on  en=off  dbl_ovrd=off  block_type=register
      settings: block_version=8.2
  Reinterpret : xbsIndex_r4/Reinterpret  force_arith_type=on  arith_type=Unsigned  force_bin_pt=off  bin_pt=0  block_type=reinterpret
      settings: infoedit="Changes signal type without altering the binary representation.   You can changed the signal between signed and unsigned, and relocate the binary point.<P><P>Hardware notes: In hardware this block costs nothing.<P><P>Example:  Suppose the input is 6 bits wide, signed, with 2 fractional bits, and the output is forced to unsigned with 0 fractional bits.  Then an input of -2.0 (1110.00 in binary 2's complement) becomes an output of 56 (111000 in binary)."  block_version=8.2
  Reinterpret1 : xbsIndex_r4/Reinterpret  force_arith_type=on  arith_type="Signed  (2's comp)"  force_bin_pt=on  bin_pt=15  block_type=reinterpret
      settings: infoedit="Changes signal type without altering the binary representation.   You can changed the signal between signed and unsigned, and relocate the binary point.<P><P>Hardware notes: In hardware this block costs nothing.<P><P>Example:  Suppose the input is 6 bits wide, signed, with 2 fractional bits, and the output is forced to unsigned with 0 fractional bits.  Then an input of -2.0 (1110.00 in binary 2's complement) becomes an output of 56 (111000 in binary)."  block_version=8.2
  Reinterpret2 : xbsIndex_r4/Reinterpret  force_arith_type=on  arith_type="Signed  (2's comp)"  force_bin_pt=on  bin_pt=15  block_type=reinterpret
      settings: infoedit="Changes signal type without altering the binary representation.   You can changed the signal between signed and unsigned, and relocate the binary point.<P><P>Hardware notes: In hardware this block costs nothing.<P><P>Example:  Suppose the input is 6 bits wide, signed, with 2 fractional bits, and the output is forced to unsigned with 0 fractional bits.  Then an input of -2.0 (1110.00 in binary 2's complement) becomes an output of 56 (111000 in binary)."  block_version=8.2
  Relational : xbsIndex_r4/Relational  mode=a=b  en=off  latency=2  dbl_ovrd=off  block_type=relational
      settings: block_version=8.2
  Slice : xbsIndex_r4/Slice  nbits=16  boolean_output=off  mode=Upper Bit Location + Width  bit1=0  base1=MSB of Input  bit0=0  base0=LSB of Input  dbl_ovrd=off  block_type=slice
      settings: infoedit="Extracts a given range of bits from each input sample and presents it at the output.  The output type is ordinarily unsigned with binary point at zero, but can be Boolean when the slice is one bit wide.<P><P>Hardware notes: In hardware this block costs nothing."  block_version=8.2
  Slice1 : xbsIndex_r4/Slice  nbits=16  boolean_output=off  mode=Lower Bit Location + Width  bit1=0  base1=MSB of Input  bit0=0  base0=LSB of Input  dbl_ovrd=off  block_type=slice
      settings: infoedit="Extracts a given range of bits from each input sample and presents it at the output.  The output type is ordinarily unsigned with binary point at zero, but can be Boolean when the slice is one bit wide.<P><P>Hardware notes: In hardware this block costs nothing."  block_version=8.2
  Wr Control : Subsystem
  I Delay Out : Outport
  Q Delay Out : Outport  Port=2
  wires:
  IQ_In/1 -> Delay/1
  Reset/1 -> FIFO/4, FIFO1/4, Logical4/2, Logical3/2
  FIFO1/1 -> Register/1
  FIFO/1 -> Register1/1, Display4/1
  Register1/1 -> Mux/2
  Register/1 -> Mux/3
  Relational/1 -> Mux/1
  Constant1/1 -> Relational/2
  Reinterpret/1 -> Relational/1
  Delay/1 -> FIFO1/1, FIFO/1, Display1/1
  Logical3/1 -> Register1/2
  Logical4/1 -> Register/2
  Inverter1/1 -> Logical4/1
  Inverter/1 -> Logical3/1
  Mux/1 -> Slice/1, Slice1/1, Display5/1
  Slice/1 -> Reinterpret2/1
  Slice1/1 -> Reinterpret1/1
  Reinterpret1/1 -> Q Delay Out/1
  Reinterpret2/1 -> I Delay Out/1
  Wr Control/1(Wr1) -> FIFO/2, Reinterpret/1, FIFO1/3, Inverter1/1, Display2/1
  Wr Control/2(Wr2) -> FIFO/3, FIFO1/2, Inverter/1, Display3/1
  Gate1/1 -> Wr Control/1(Gate1)
  Gate2/1 -> Wr Control/2(Gate2)

== system PulsePairProc_x4/Pulse Pair Processor D/Calc/I^2+Q^2 ==
  I : Inport
  Q : Inport  Port=2
  AddSub : xbsIndex_r4/AddSub  mode=Addition  use_carryin=off  use_carryout=off  en=off  latency=1  precision=User Defined  arith_type=Unsigned  n_bits=32  bin_pt=32  quantization="Round  (unbiased: +/- Inf)"  overflow=Flag as error  dbl_ovrd=off  use_behavioral_HDL=off  pipelined=on  use_rpm=on  block_type=addsub
      settings: block_version=8.2
  Mult : xbsIndex_r4/Mult  precision=User Defined  arith_type=Unsigned  n_bits=32  bin_pt=32  quantization="Round  (unbiased: +/- Inf)"  overflow=Flag as error  en=off  latency=1  dbl_ovrd=off  use_behavioral_HDL=off  use_embedded=on  optimum_pipeline=off  use_rpm=on  placement_style=Rectangular shape  pipeline=on  block_type=mult
      settings: infoedit=Hardware notes: To use the internal pipeline stage of the dedicated multiplier you must select 'Pipeline for maximum performance'.  block_version=8.2
  Mult1 : xbsIndex_r4/Mult  precision=User Defined  arith_type=Unsigned  n_bits=32  bin_pt=32  quantization="Round  (unbiased: +/- Inf)"  overflow=Flag as error  en=off  latency=1  dbl_ovrd=off  use_behavioral_HDL=off  use_embedded=on  optimum_pipeline=off  use_rpm=on  placement_style=Rectangular shape  pipeline=on  block_type=mult
      settings: infoedit=Hardware notes: To use the internal pipeline stage of the dedicated multiplier you must select 'Pipeline for maximum performance'.  block_version=8.2
  P : Outport
  wires:
  Mult/1 -> AddSub/1
  Mult1/1 -> AddSub/2
  I/1 -> Mult/1, Mult/2
  Q/1 -> Mult1/1, Mult1/2
  AddSub/1 -> P/1

== system PulsePairProc_x4/Pulse Pair Processor D/Calc/Q*Id1-I*Qd1 ==
  Q : Inport
  I Delay 1 : Inport  Port=2
  I : Inport  Port=3
  Q Delay 1 : Inport  Port=4
  AddSub2 : xbsIndex_r4/AddSub  mode=Subtraction  use_carryin=off  use_carryout=off  en=off  latency=1  precision=User Defined  arith_type="Signed  (2's comp)"  n_bits=32  bin_pt=31  quantization="Round  (unbiased: +/- Inf)"  overflow=Flag as error  dbl_ovrd=off  use_behavioral_HDL=off  pipelined=on  use_rpm=on  block_type=addsub
      settings: block_version=8.2
  Mult4 : xbsIndex_r4/Mult  precision=User Defined  arith_type="Signed  (2's comp)"  n_bits=32  bin_pt=31  quantization="Round  (unbiased: +/- Inf)"  overflow=Saturate  en=off  latency=1  dbl_ovrd=off  use_behavioral_HDL=off  use_embedded=on  optimum_pipeline=off  use_rpm=on  placement_style=Rectangular shape  pipeline=on  block_type=mult
      settings: infoedit=Hardware notes: To use the internal pipeline stage of the dedicated multiplier you must select 'Pipeline for maximum performance'.  block_version=8.2
  Mult5 : xbsIndex_r4/Mult  precision=User Defined  arith_type="Signed  (2's comp)"  n_bits=32  bin_pt=31  quantization="Round  (unbiased: +/- Inf)"  overflow=Saturate  en=off  latency=1  dbl_ovrd=off  use_behavioral_HDL=off  use_embedded=on  optimum_pipeline=off  use_rpm=on  placement_style=Rectangular shape  pipeline=on  block_type=mult
      settings: infoedit=Hardware notes: To use the internal pipeline stage of the dedicated multiplier you must select 'Pipeline for maximum performance'.  block_version=8.2
  B : Outport
  wires:
  Mult4/1 -> AddSub2/1
  Mult5/1 -> AddSub2/2
  Q/1 -> Mult4/1
  I Delay 1/1 -> Mult4/2
  AddSub2/1 -> B/1
  I/1 -> Mult5/1
  Q Delay 1/1 -> Mult5/2

== system PulsePairProc_x4/Pulse Pair Processor D/Sum/A Avg ==
  A_Data_In : Inport
  M : Inport  Port=2
  N : Inport  Port=3
  Gate 1 : Inport  Port=4
  Gate 2 : Inport  Port=5
  Reset : Inport  Port=6
  Avg. A 1 : Subsystem
  Avg. A 2 : Subsystem
  A1 : Outport
  A2 : Outport  Port=2
  ABP G1 : Outport  Port=3
  ABP G2 : Outport  Port=4
  wires:
  A_Data_In/1 -> Avg. A 1/1(In), Avg. A 2/1(In)
  M/1 -> Avg. A 1/2(M), Avg. A 2/2(M)
  N/1 -> Avg. A 1/3(N), Avg. A 2/3(N)
  Avg. A 1/1(Out) -> A1/1
  Gate 1/1 -> Avg. A 1/4(Gate)
  Avg. A 2/1(Out) -> A2/1
  Gate 2/1 -> Avg. A 2/4(Gate)
  Avg. A 1/2(A,B,P Gate 1) -> ABP G1/1
  Avg. A 2/2(A,B,P Gate 1) -> ABP G2/1
  Reset/1 -> Avg. A 1/5(Reset), Avg. A 2/5(Reset)
